simulink model "propeller"  (R2020b)
settings: Solver=VariableStepAuto  StartTime=0.0  StopTime=10.0  RelTol=1e-3
model mask{D=11, Ct=[1 0], Cp=[1 0]}
  mask prompts: D "Propeller Diameter [in]:"; Ct "Coefficient of Thrust Advance Ratio Polynomial:"; Cp "Coefficient of Power Advance Ratio Polynomial:"
model workspace (MAT data in the model file):
  Cp = Simulink.Parameter
  Cp.Value = [1 0]
  Cp.DataType = 'auto'
  Cp.Dimensions = [1 2]
  Ct = Simulink.Parameter
  Ct.Value = [1 0]
  Ct.DataType = 'auto'
  Ct.Dimensions = [1 2]
  D = Simulink.Parameter
  D.Value = 11
  D.DataType = 'auto'
  D.Dimensions = [1 1]
libraries: aerolibconvert2 x3
settings Model: ParameterArgumentNames=Cp,Ct,D  OrderedModelArguments=off  Creator=brian  LastModifiedBy=brian

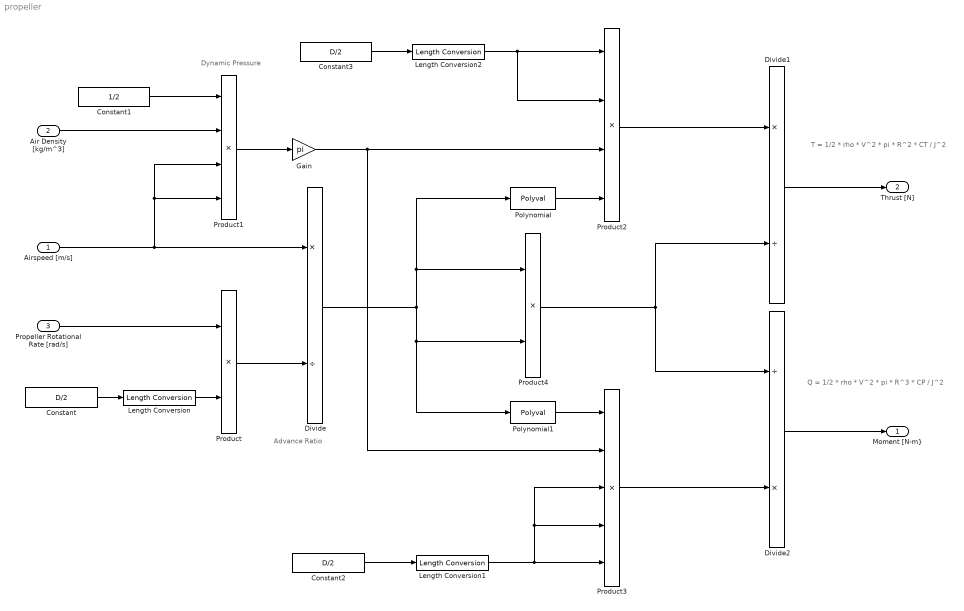
== system propeller ==
  note: Q = 1/2 * rho * V^2 * pi * R^3 * CP / J^2
  note: T = 1/2 * rho * V^2 * pi * R^2 * CT / J^2
  note: Dynamic Pressure
  note: Advance Ratio
  Airspeed [m/s] : Inport
  Air Density [kg/m^3] : Inport  Port=2
  Propeller Rotational Rate [rad/s] : Inport  Port=3
  Constant : Constant  Value=D/2
  Constant1 : Constant  Value=1/2
  Constant2 : Constant  Value=D/2
  Constant3 : Constant  Value=D/2
  Divide : Product  Inputs=*/
  Divide1 : Product  Inputs=*/
  Divide2 : Product  Inputs=/*
  Gain : Gain  Gain=pi
  Length Conversion : aerolibconvert2/Length Conversion  IU=in  OU=m
  Length Conversion1 : aerolibconvert2/Length Conversion  IU=in  OU=m
  Length Conversion2 : aerolibconvert2/Length Conversion  IU=in  OU=m
  Polynomial : Polyval  Coefs=Ct
  Polynomial1 : Polyval  Coefs=Cp
  Product : Product
  Product1 : Product  Inputs=4
  Product2 : Product  Inputs=4
  Product3 : Product  Inputs=5
  Product4 : Product
  "Moment [N-m}" : Outport
  Thrust [N] : Outport  Port=2
  wires:
  Airspeed [m/s]/1 -> Divide/1, Product1/4, Product1/3
  Propeller Rotational Rate [rad/s]/1 -> Product/1
  Product/1 -> Divide/2
  Constant/1 -> Length Conversion/1
  Air Density [kg/m^3]/1 -> Product1/2
  Constant1/1 -> Product1/1
  Divide/1 -> Product4/2, Polynomial1/1, Product4/1, Polynomial/1
  Product1/1 -> Gain/1
  Polynomial/1 -> Product2/4
  Polynomial1/1 -> Product3/1
  Gain/1 -> Product3/2, Product2/3
  Constant2/1 -> Length Conversion1/1
  Constant3/1 -> Length Conversion2/1
  Product3/1 -> Divide2/2
  Product2/1 -> Divide1/1
  Product4/1 -> Divide2/1, Divide1/2
  Divide1/1 -> Thrust [N]/1
  Divide2/1 -> "Moment [N-m}"/1
  Length Conversion/1 -> Product/2
  Length Conversion1/1 -> Product3/4, Product3/3, Product3/5
  Length Conversion2/1 -> Product2/2, Product2/1
